simulink model "Receiver_Assignmet_2"  (R2023b)
settings: Solver=FixedStepAuto  StartTime=0.0  StopTime=10.0  RelTol=1e-3
undefined symbols (not defined in the file): Data_Display, enable_decrypt, key, method, Seed, tx_2
libraries: androiduilib x5, androidaudiovideolib x1, androidcommunicationlib x1
settings Model: Creator=krish  LastModifiedBy=krish
settings OptimizationCC: EnhancedBackFolding=on  PassReuseOutputArgsAs=Individual arguments  ZeroExternalMemoryAtStartup=off  ZeroInternalMemoryAtStartup=off  MaxStackSize=64  OptimizeBlockOrder=speed  DifferentSizesBufferReuse=on  OptimizationCustomize=off  EfficientTunableParamExpr=on
settings DebuggingCC: ParameterTunabilityLossMsg=error
settings HardwareCC: ProdBitPerLong=64  ProdLargestAtomicInteger=LongLong  ProdLargestAtomicFloat=Double  ProdLongLongMode=on  ProdHWDeviceType=ARM Compatible->ARM 64-bit (LP64)  UseEmbeddedCoderFeatures=off  UseSimulinkCoderFeatures=off
settings SFSimCC: MATLABDynamicMemAlloc=off
settings RTWCC: Description=Embedded Coder  SystemTargetFile=ert.tlc  HardwareBoard=Android Device (64bit)  TLCOptions="-aInlineSetEventsForThisBaseRateFcn=TLC_FALSE -aSuppressMultiTaskScheduler=TLC_FALSE  -aRateBasedStepFcn=0"  TemplateMakefile=ert_default_tmf  RTWVerbose=off  Toolchain=Android SDK/NDK Tools
settings CodeAppCC: ForceParamTrailComments=on  IgnoreCustomStorageClasses=off  OperatorAnnotations=on  SimulinkDataObjDesc=on  SFDataObjDesc=on  InsertBlockDesc=on
settings ERTTargetCC: SupportNonInlinedSFcns=on

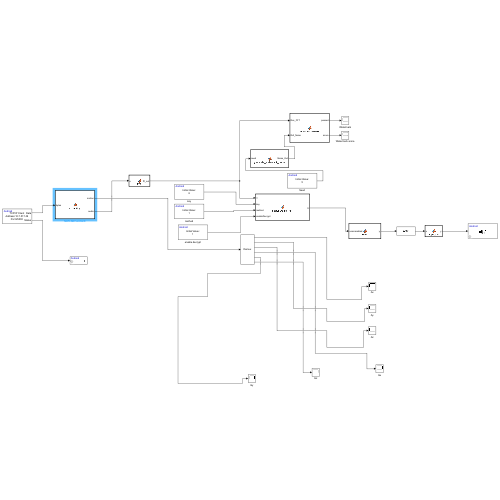
[thumbnail: Simulink's stored preview of the top-level diagram]
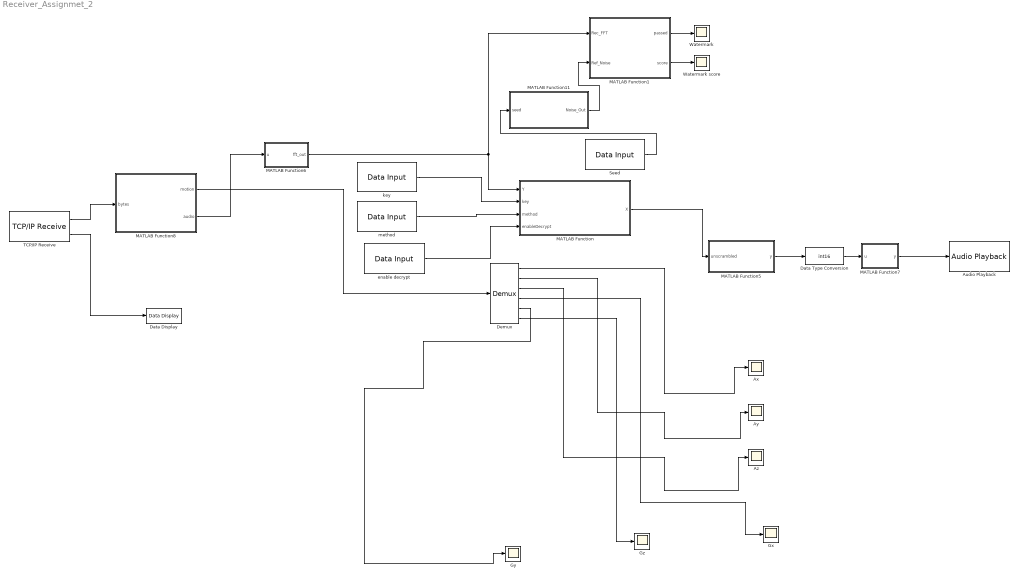
== system Receiver_Assignmet_2 ==
  Audio Playback : androidaudiovideolib/Audio Playback  SampleFreq=44100  AudioSamplingFreq=44100  SampleTime=0.1  DeviceStr=0  QueueDuration=0  BlockPlatform=Android
  Ax : Scope
  Ay : Scope
  Az : Scope
  Data Display : androiduilib/Data Display  DataDisplayId=tx_2/Data_Display  Format=Float  Precision=6  SimulateUsing=Code generation  blockPlatform=Android
  Data Type Conversion : DataTypeConversion  OutDataTypeStr=int16  SaturateOnIntegerOverflow=off  RndMeth=Floor
  Demux : Demux  Outputs=6
      settings: DisplayOption=none
  Gx : Scope
  Gy : Scope
  Gz : Scope
  MATLAB Function : MATLAB Function  TreatAsAtomicUnit=on
  MATLAB Function1 : MATLAB Function  TreatAsAtomicUnit=on
  MATLAB Function11 : MATLAB Function  TreatAsAtomicUnit=on
  MATLAB Function5 : MATLAB Function  TreatAsAtomicUnit=on
  MATLAB Function6 : MATLAB Function  TreatAsAtomicUnit=on
  MATLAB Function7 : MATLAB Function  TreatAsAtomicUnit=on
  MATLAB Function8 : MATLAB Function  TreatAsAtomicUnit=on
  Seed : androiduilib/Data Input  isCharVector=off  Value=5  CharVector=Hello World  OutputDataType=double  maxCharVectorSize=100  DataInputId=tx_2/Seed  SampleTime=0.1
  TCP/IP Receive : androidcommunicationlib/TCP//IP Receive  TCPReceiveId=tx_2/TCP//IP_Receive  Mode_=Client  LocalServerPort_=25000  RemoteAddr_=10.7.57.149  RemoteServerPort_=25000  DataType_=uint8  DataSize_=8844  SampleTime_=0.1  ClientPortBindingSelection_=off  ClientPortToBind_=35000  BlockingMode_=on  BlockTimeout_=0.1
  Watermark : Scope
  Watermark score : Scope
  enable decrypt : androiduilib/Data Input  isCharVector=off  Value=1.0  CharVector=Hello World  OutputDataType=double  maxCharVectorSize=100  DataInputId=tx_2/enable_decrypt  SampleTime=0.1
  key : androiduilib/Data Input  isCharVector=off  Value=6  CharVector=Hello World  OutputDataType=double  maxCharVectorSize=100  DataInputId=tx_2/key  SampleTime=0.1
  method : androiduilib/Data Input  isCharVector=off  Value=1.0  CharVector=Hello World  OutputDataType=double  maxCharVectorSize=100  DataInputId=tx_2/method  SampleTime=0.1
  wires:
  MATLAB Function11/1(Noise_Out) -> MATLAB Function1/2(Ref_Noise)
  Demux/1 -> Ax/1
  Demux/3 -> Az/1
  MATLAB Function8/2(audio) -> MATLAB Function6/1(u)
  key/1 -> MATLAB Function/2(key)
  Demux/4 -> Gx/1
  method/1 -> MATLAB Function/3(method)
  MATLAB Function/1(X) -> MATLAB Function5/1(unscrambled)
  Demux/2 -> Ay/1
  MATLAB Function5/1(y) -> Data Type Conversion/1
  MATLAB Function8/1(motion) -> Demux/1
  MATLAB Function6/1(fft_out) -> MATLAB Function/1(Y), MATLAB Function1/1(Rec_FFT)
  Demux/5 -> Gy/1
  Demux/6 -> Gz/1
  Data Type Conversion/1 -> MATLAB Function7/1(u)
  MATLAB Function7/1(y) -> Audio Playback/1
  MATLAB Function1/2(score) -> Watermark score/1
  MATLAB Function1/1(passed) -> Watermark/1
  Seed/1 -> MATLAB Function11/1(seed)
  enable decrypt/1 -> MATLAB Function/4(enableDecrypt)
  TCP/IP Receive/2 -> Data Display/1
  TCP/IP Receive/1 -> MATLAB Function8/1(bytes)

== matlab function Receiver_Assignmet_2/MATLAB Function1 ==
  data: Rec_FFT input; passed output; Ref_Noise input; score output
function [passed, score] = verify_watermark(Rec_FFT, Ref_Noise)

    persistent latched_state;

    if isempty(latched_state)
        latched_state = false;
    end

    THRESHOLD = 0.15;
    MIN_ENERGY = 0.0001;

    R = double(Rec_FFT(:));
    N = double(Ref_Noise(:));
    
    if isempty(R) || isempty(N)
        passed = latched_state; 
        score = 0; 
        return;
    end

    mask_indices = abs(N) > 0;
    
    if sum(mask_indices) == 0
        passed = latched_state; 
        score = 0; 
        return;
    end
    
    R_band = R(mask_indices);
    N_band = N(mask_indices);

    E_sig   = sum(abs(R_band).^2);
    E_noise = sum(abs(N_band).^2);
    
    if E_sig < MIN_ENERGY
        passed = latched_state; 
        score = 0;
        return;
    end

    corr_val = abs(sum(R_band .* conj(N_band)));
    
    denominator = sqrt(E_sig * E_noise);
    
    if denominator < 1e-12
        score = 0;
    else
        score = corr_val / denominator;
    end

    if score > THRESHOLD
        latched_state = true;
    end
    
    passed = latched_state;

end

== matlab function Receiver_Assignmet_2/MATLAB Function ==
  data: Y input; X output; key input; method input; enableDecrypt input
function X = decryptAudio_FFT(Y, key, method, enableDecrypt)

    [N, C] = size(Y);
    X = complex(zeros(N, C, 'like', Y));
    
    if nargin < 4 || enableDecrypt == 0
        X = Y; return;
    end
    
    if ischar(key) || isstring(key)
        keyChar = double(char(key));
        keynum = sum(keyChar .* (1:length(keyChar))); 
    else
        keynum = double(key);
    end
    seedVal = max(1, floor(abs(keynum)));

    switch int16(method)
        
        % CASE 1: Unscramble
        case 1
            X = keyUnscrambleFFT(Y, seedVal);

        % CASE 2: Remove Adaptive Spectrum Noise
        case 2
            s = rng;
            rng(seedVal, 'twister');

            magY = abs(Y);
            magEnv = movmean(magY, 8, 1);

            noise_white = randn(N, C);
            f_bins = (1:N)';
            pink_filter = 1 ./ (sqrt(f_bins) + 1);
            noise_pink = noise_white .* pink_filter;

            normalized_env = magEnv ./ max(magEnv(:) + eps);
            noise_adaptive = noise_pink .* normalized_env;

            noise_level = 1000 * mean(magY(:)); 
            noise_final = noise_adaptive * noise_level;

            magRec = magY - abs(noise_final);
            magRec(magRec < 0) = 0;

            phaseY = angle(Y);
            X = magRec .* exp(1j * phaseY);

            rng(s);

            
        % CASE 3: WaterMark (No use here so we let the signal pass)
        case 3
            X = Y; 
            
        otherwise
            X = Y;
    end
end

function X = keyUnscrambleFFT(Y, key)
    [N, C] = size(Y);
    posIdx = 2:floor(N/2);
    negIdx = N - posIdx + 2;
    K = numel(posIdx);
    if K == 0; X = Y; return; end
    b = mod(key, K); a = mod(key, K-1) + 1;
    while K > 1 && gcd(a, K) ~= 1; a = a + 1; if a >= K; a = 1; end; end
    [g, inv_a, ~] = gcd(a, K); inv_a = mod(inv_a, K);
    inv_perm = zeros(1, K);
    for m = 1:K; inv_perm(m) = mod(inv_a * ((m-1) - b), K) + 1; end
    if ~isreal(Y); X = complex(zeros(N, C, 'like', Y)); else; X = zeros(N, C, 'like', Y); end
    X(1, :) = Y(1, :);
    if mod(N,2) == 0; X(N/2 + 1, :) = Y(N/2 + 1, :); end
    X(posIdx, :) = Y(posIdx(inv_perm), :);
    if ~isreal(Y); X(negIdx, :) = conj(X(posIdx, :)); else; X(negIdx, :) = X(posIdx, :); end
end

== matlab function Receiver_Assignmet_2/MATLAB Function5 ==
  data: unscrambled input; y output
function y = IFFT(unscrambled)
    N = length(unscrambled);
    unscrambled(2:N/2) = conj(unscrambled(N:-1:N/2+2));
    Channel = ifft(unscrambled);
    y = real(Channel);
end

== matlab function Receiver_Assignmet_2/MATLAB Function6 ==
  data: u input; fft_out output
function fft_out = FFT(u)
    u = u(:,1);
    fft_out = fft(u);
end

== matlab function Receiver_Assignmet_2/MATLAB Function7 ==
  data: u input; y output
function y = duplicate(u)
y = [u, u];

== matlab function Receiver_Assignmet_2/MATLAB Function8 ==
  data: bytes input; motion output; audio output
function [motion, audio] = unpacking(bytes)
                 
motion = zeros(1,6,'single');         % 1x6
audio = zeros(4410,1,'int16');       % 4410x1


motion(1,1:6)  = typecast(bytes(1:24), 'single').';   % 6 singles
audio(:,1)  = typecast(bytes(25:8844), 'int16');   % 4410 samples
end

== matlab function Receiver_Assignmet_2/MATLAB Function11 ==
  data: seed input; Noise_Out output
function Noise_Out = generate_watermark_noise(seed)
    N = 4410; 
    Fs = 44100;
    df = Fs / N;
    f_start_hz = 200;
    f_end_hz   = 10000;
    
    alpha = 5000; 

    idx_start = floor(f_start_hz / df) + 1;
    idx_end   = ceil(f_end_hz / df) + 1;
    
    if idx_end > (N/2)
        idx_end = floor(N/2);
    end

    rng(uint32(seed), 'twister');
    
    num_bins = idx_end - idx_start + 1;

    noise_real = randn(num_bins, 1);
    noise_imag = randn(num_bins, 1);
    
    noise_band = alpha * complex(noise_real, noise_imag);

    Noise_Out = complex(zeros(N, 1));
    
    current_bin = 0;
    for i = idx_start : idx_end
        current_bin = current_bin + 1;
        Noise_Out(i) = noise_band(current_bin);
    end

    current_bin = 0;
    for k = idx_start : idx_end
        current_bin = current_bin + 1;
        mirror_idx = N - k + 2;
        
        if mirror_idx <= N
            Noise_Out(mirror_idx) = conj(noise_band(current_bin));
        end
    end

end
